simulink model "rtwdemo_condinput"  (Simulink 7.6)
settings: Solver=FixedStepDiscrete  StartTime=0.0  StopTime=500  RelTol=1e-3  SampleTimeConstraint=STIndependent
libraries: rtwdemowidgets x2
Description:
  | Conditional Input Branch Execution
settings Model: Creator=The MathWorks Inc.  ExtModeAutoUpdateStatusClock=off
settings DataIOCC: SaveOutput=off  SaveTime=off  SignalLoggingName=sigsOut
settings OptimizationCC: InlineParams=on  InlineInvariantSignals=on  StateBitsets=on  DataBitsets=on  UseTempVars=on  EfficientFloat2IntCast=on  EfficientMapNaN2IntZero=off
settings DebuggingCC: CheckExecutionContextPreStartOutputMsg=on  CheckExecutionContextRuntimeOutputMsg=on  SolverPrmCheckMsg=none  StrictBusMsg=ErrorOnBusTreatedAsVector
settings HardwareCC: ProdIntDivRoundTo=Zero  ProdEndianess=LittleEndian  ProdHWDeviceType=Generic->32-bit Embedded Processor  TargetHWDeviceType=Generic->32-bit Embedded Processor
settings RTWCC: TLCOptions=-p0 -aWarnNonSaturatedBlocks=0  GenerateReport=on  RTWVerbose=off  ProcessScript=grt_make_rtw_hook  LaunchReport=on
settings CodeAppCC: ForceParamTrailComments=on
settings GRTTargetCC: TargetFcnLib=ansi_tfl_tmw.mat

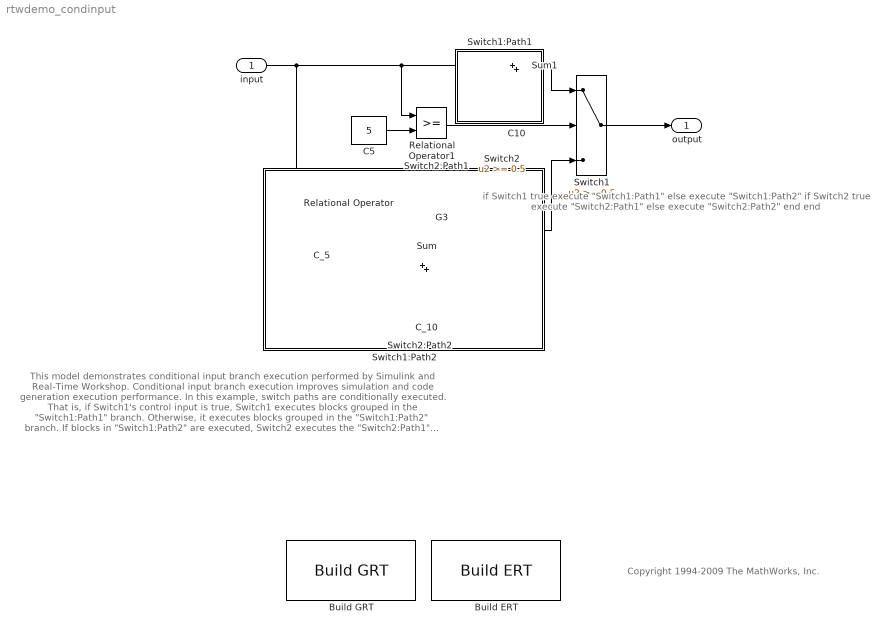
== system rtwdemo_condinput ==
  note: if Switch1 true
      |    execute "Switch1:Path1"
      |  else
      |    execute "Switch1:Path2"
      |    if Switch2 true
      |      execute "Switch2:Path1"
      |    else
      |      execute "Switch2:Path2"
      |    end
      |  end
  note: This model demonstrates conditional input branch execution performed by Simulink and
      | Real-Time Workshop. Conditional input branch execution improves simulation and code
      | generation execution performance. In this example, switch paths are conditionally executed.
      | That is, if Switch1's control input is true, Switch1 executes blocks grouped in the
      | "Switch1:Path1" branch. Otherwise, it executes blocks grouped in the "Switch1:Path2" branch.
      | If blocks in "Switch1:Path2" are executed, Switch2 executes the "Switch2:Path1" branch if
      | its control input is true.  Otherwise, it executes the "Switch2:Path2" branch.  This logic
      | is illustrated by the pseudo code above.
  note: Copyright 1994-2009 The MathWorks, Inc.
  input : Inport  OutDataTypeStr=double  PortDimensions=1
  "  C10" : Constant  Value=10
  "  G3" : Gain  Gain=3  SaturateOnIntegerOverflow=on  OutDataTypeStr=Inherit: Same as input  ParamDataTypeStr=Inherit: Same as input
  " C_10" : Constant  Value=-10
  " Sum" : Sum  Inputs=|++  SaturateOnIntegerOverflow=on  InputSameDT=on  OutDataTypeStr=Inherit: Same as first input
  " Sum1" : Sum  Inputs=|++  SaturateOnIntegerOverflow=on  InputSameDT=on  OutDataTypeStr=Inherit: Same as first input
  " Switch2" : Switch  Threshold=0.5  SaturateOnIntegerOverflow=on  InputSameDT=on
  " Switch2:Path1" : Subsystem
      settings: AttributesFormatString=\n  OpenFcn=disp('');
      mask Display: disp(' ')
  " Switch2:Path2" : Subsystem
      settings: AttributesFormatString=\n  OpenFcn=disp('');
      mask Display: disp(' ')
  Build ERT : rtwdemowidgets/Build ERT  SystemSampleTime=-1  attrib_overrides={}
  Build GRT : rtwdemowidgets/Build GRT  SystemSampleTime=-1  attrib_overrides={}
  C5 : Constant  Value=5
  C_5 : Constant  Value=-5
  Relational Operator : RelationalOperator  InputSameDT=on
  Relational Operator1 : RelationalOperator  InputSameDT=on
  Switch1 : Switch  Threshold=0.5  SaturateOnIntegerOverflow=on  InputSameDT=on
  Switch1:Path1 : Subsystem
      settings: AttributesFormatString=\n  OpenFcn=disp('');
      mask Display: disp(' ')
  Switch1:Path2 : Subsystem
      settings: AttributesFormatString=\n  OpenFcn=disp('');
      mask Display: disp(' ')
  output : Outport
  wires:
  Relational Operator/1 -> " Switch2"/2
  " Switch2"/1 -> Switch1/3
  input/1 -> " Sum"/1, Relational Operator/1, "  G3"/1, Relational Operator1/1, " Sum1"/1
  "  G3"/1 -> " Switch2"/1
  " Sum1"/1 -> Switch1/1
  " Sum"/1 -> " Switch2"/3
  C5/1 -> Relational Operator1/2
  C_5/1 -> Relational Operator/2
  Switch1/1 -> output/1
  " C_10"/1 -> " Sum"/2
  "  C10"/1 -> " Sum1"/2
  Relational Operator1/1 -> Switch1/2

== system rtwdemo_condinput/ Switch2:Path1 ==

== system rtwdemo_condinput/ Switch2:Path2 ==

== system rtwdemo_condinput/Switch1:Path1 ==

== system rtwdemo_condinput/Switch1:Path2 ==
